simulink model "mA2_vessel"  (R2023a)
settings: Solver=ode4  StartTime=0.0  StopTime=50  FixedStep=0.01  RelTol=1e-3
values from neighbouring files (symbols this model uses):
  B_vessel = 0    [init_mA2_vessel.m]
  d_quay = 0    [init_mA2_vessel.m]
  initial_position = [0,0,0,0,0,0]'    [init_mA2_vessel.m]
  initial_velocity = [0,0,0,0,0,0]'    [init_mA2_vessel.m]
  k_quay = 0    [init_mA2_vessel.m]
  L_vessel = 0    [init_mA2_vessel.m]
  mu_quay = 0    [init_mA2_vessel.m]
  quay_1_depth = 0    [init_mA2_vessel.m]
  quay_1_en = false    [init_mA2_vessel.m]
  quay_1_p0 = [0, 0]'    [init_mA2_vessel.m]
  quay_1_p1 = [0, 0]'    [init_mA2_vessel.m]
  quay_2_depth = 0    [init_mA2_vessel.m]
  quay_2_en = false    [init_mA2_vessel.m]
  quay_2_p0 = [0, 0]'    [init_mA2_vessel.m]
  quay_2_p1 = [0, 0]'    [init_mA2_vessel.m]
  quay_3_depth = 0    [init_mA2_vessel.m]
  quay_3_en = false    [init_mA2_vessel.m]
  quay_3_p0 = [0, 0]'    [init_mA2_vessel.m]
  quay_3_p1 = [0, 0]'    [init_mA2_vessel.m]
  quay_4_depth = 0    [init_mA2_vessel.m]
  quay_4_en = false    [init_mA2_vessel.m]
  quay_4_p0 = [0, 0]'    [init_mA2_vessel.m]
  quay_4_p1 = [0, 0]'    [init_mA2_vessel.m]
libraries: mssSimulink x2
settings Model: Creator=tobiasvt  LastModifiedBy=HalvorPlatou
settings SolverCC: AlgebraicLoopSolver=TrustRegion
settings DebuggingCC: UnconnectedInputMsg=warning  UnconnectedOutputMsg=warning  UnconnectedLineMsg=warning
settings ModelReferenceCC: EnableRefExpFcnMdlSchedulingChecks=on
settings SFSimCC: CustomCodeUndefinedFunction=UseInterfaceOnly
settings RTWCC: Description=FMU based on GRT (Functional Mock-up Unit)  SystemTargetFile=grtfmi.tlc  GenerateMakefile=off  TemplateMakefile=none  RetainRTWFile=on  DLArmComputeVersion=19.05
settings STFCustomTargetCC: ConcurrentExecutionCompliant=off  CombineOutputUpdateFcns=on  CodeInterfacePackaging=Reusable function  GRTInterface=off  GenerateAllocFcn=on  UseToolchainInfoCompliant=off  SystemTargetFile=grtfmi.tlc
settings GRTTargetCC: ParMdlRefBuildCompliant=off  CompOptLevelCompliant=off  ConcurrentExecutionCompliant=off  MatFileLogging=off  CodeInterfacePackaging=Reusable function  CPPClassGenCompliant=off  GenerateAllocFcn=on  UseToolchainInfoCompliant=off

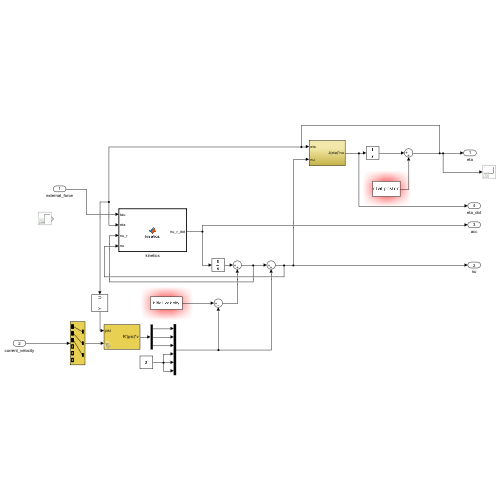
[thumbnail: Simulink's stored preview of the top-level diagram]
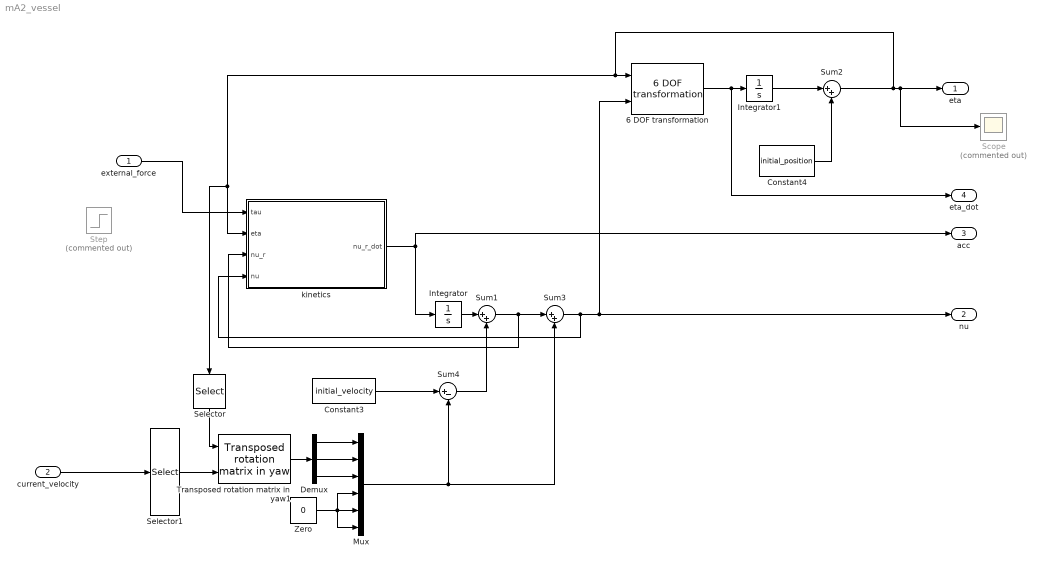
== system mA2_vessel ==
  external_force : Inport  PortDimensions=6
  current_velocity : Inport  Port=2  PortDimensions=6
  6 DOF transformation : mssSimulink/Modelling/Kinematics/6 DOF transformation  SystemSampleTime=-1  VariantActivationTime=update diagram  Latency=0  AutoFrameSizeCalculation=off
  Constant3 : Constant  Value=initial_velocity
  Constant4 : Constant  Value=initial_position
  Demux : Demux  Outputs=3
  Integrator : Integrator
  Integrator1 : Integrator
  Mux : Mux  Inputs=6
  Scope : Scope  Commented=on
  Selector : Selector  InputPortWidth=6  IndexOptions=Index vector (dialog)  Indices=[6]  OutputSizes=1
  Selector1 : Selector  InputPortWidth=6  IndexOptions=Index vector (dialog)  Indices=[1 2 3]  OutputSizes=1
  Step : Step  Commented=on  Before=[0,0,0,0,0,0]  After=[1000,0,0,0,0,0]  SampleTime=0
  Sum1 : Sum  Inputs=|++
  Sum2 : Sum  Inputs=|++
  Sum3 : Sum  Inputs=|++
  Sum4 : Sum  Inputs=|+-
  Transposed rotation matrix in yaw1 : mssSimulink/Modelling/Kinematics/Transposed rotation  matrix in yaw
  Zero : Constant  Value=0  OutDataTypeStr=Inherit: Inherit via back propagation
  kinetics : MATLAB Function  TreatAsAtomicUnit=on
  eta : Outport  VectorParamsAs1DForOutWhenUnconnected=off
  nu : Outport  Port=2  VectorParamsAs1DForOutWhenUnconnected=off
  acc : Outport  Port=3  VectorParamsAs1DForOutWhenUnconnected=off
  eta_dot : Outport  Port=4  VectorParamsAs1DForOutWhenUnconnected=off
  wires:
  Demux/1 -> Mux/1
  Sum1/1 -> kinetics/3(nu_r), Sum3/1
  Demux/3 -> Mux/3
  Selector1/1 -> Transposed rotation matrix in yaw1/2
  Sum2/1 -> 6 DOF transformation/1, Selector/1, kinetics/2(eta), Scope/1, eta/1
  Mux/1 -> Sum4/2, Sum3/2
  Demux/2 -> Mux/2
  kinetics/1(nu_r_dot) -> acc/1, Integrator/1
  Transposed rotation matrix in yaw1/1 -> Demux/1
  Integrator/1 -> Sum1/1
  Zero/1 -> Mux/6, Mux/4, Mux/5
  Constant4/1 -> Sum2/2
  Sum3/1 -> kinetics/4(nu), 6 DOF transformation/2, nu/1
  Selector/1 -> Transposed rotation matrix in yaw1/1
  Integrator1/1 -> Sum2/1
  Constant3/1 -> Sum4/1
  Sum4/1 -> Sum1/2
  6 DOF transformation/1 -> eta_dot/1, Integrator1/1
  current_velocity/1 -> Selector1/1
  external_force/1 -> kinetics/1(tau)

== matlab function mA2_vessel/kinetics ==
  data: tau input; eta input; nu_r_dot output; nu_r input; nu input; mu_quay parameter; d_quay parameter; k_quay parameter; B_vessel parameter; L_vessel parameter; quay_1_en parameter; quay_1_depth parameter; quay_1_p1 parameter; quay_1_p0 parameter; quay_2_en parameter; quay_2_depth parameter; quay_2_p1 parameter; quay_2_p0 parameter; quay_3_en parameter; quay_3_depth parameter; quay_3_p1 parameter; quay_3_p0 parameter; quay_4_en parameter; quay_4_depth parameter; quay_4_p1 parameter; quay_4_p0 parameter
function nu_r_dot  = kinetics(tau, eta, nu_r, nu, mu_quay, d_quay, k_quay, B_vessel, L_vessel, quay_1_en, quay_1_depth, quay_1_p1, quay_1_p0, quay_2_en, quay_2_depth, quay_2_p1, quay_2_p0, quay_3_en, quay_3_depth, quay_3_p1, quay_3_p0, quay_4_en, quay_4_depth, quay_4_p1, quay_4_p0)
% Construct quay parameters
num_quays = sum([quay_1_en, quay_2_en, quay_3_en, quay_4_en]);
s = struct('line', {nan(2, 2)}, 'depth', {nan});
quays = repmat(s,1,num_quays);

i = 1;

if quay_1_en
    quays(i).line = [reshape(quay_1_p0,2,1), reshape(quay_1_p1,2,1)];
    quays(i).depth = quay_1_depth;
    i = i+1;
end
if quay_2_en
    quays(i).line = [reshape(quay_2_p0,2,1), reshape(quay_2_p1,2,1)];
    quays(i).depth = quay_2_depth;
    i = i+1;
end
if quay_3_en
    quays(i).line = [reshape(quay_3_p0,2,1), reshape(quay_3_p1,2,1)];
    quays(i).depth = quay_3_depth;
    i = i+1;
end
if quay_4_en
    quays(i).line = [reshape(quay_4_p0,2,1), reshape(quay_4_p1,2,1)];
    quays(i).depth = quay_4_depth;
    i = i+1;
end

par.mu = mu_quay;
par.k = k_quay;
par.d = d_quay;
par.v_static = 0.1;
par.stiction_damping = true;
par.vessel_polygon = [
    [L_vessel/2, B_vessel/2]
    [L_vessel/2, -B_vessel/2]
    [-L_vessel/2, -B_vessel/2]
    [-L_vessel/2, B_vessel/2]
]';

% Kinetics
u = nu_r(1);
v = nu_r(2);
r = nu_r(6);

%% Horizontal kinetics
%Hydrodynamic coefficients
m_11 = 6.8919e+03;
m_22 = 7.0591e+03;
m_33 = 3.8634e+04;
X_u = -238.5842;
X_auu = -37.1570;
X_uuu = -50.4657;
Y_v = -65.8904;
Y_avv = -300.3485;
Y_vvv = -1.8040;
Y_arv = -4.3745e+03;
Y_r = 232.5028;
Y_avr = 1.4092e+03;
Y_arr = -948.7467;
Y_ur = 223.7115;
N_v = 27.2702;
N_avv = -12.5495;
N_arv = 2.0957e+03;
N_r = -880.0850;
N_arr = -6.6088e+03;
N_avr = -583.9914;
N_uv = -262.3232;
N_ur = 854.4464;

%Mass matrix
M = [m_11 0.0 0.0;
    0.0 m_22 0.0;
    0.0 0.0 m_33];

%Damping matrix
d_11 = -X_u - X_auu*abs(u) - X_uuu*u^2;
d_22 = -Y_v - Y_avv*abs(v) - Y_arv*abs(r) - Y_vvv*v^2;
d_23 = -Y_r - Y_avr*abs(v) - Y_arr*abs(r) - Y_ur*u;
d_32 = -N_v - N_avv*abs(v) - N_arv*abs(r) - N_uv*u;
d_33 = -N_r - N_avr*abs(v) - N_arr*abs(r) - N_ur*u;

D = [d_11, 0, 0;
    0, d_22, d_23;
    0, d_32, d_33];

%Coriolis matrix
c_13 =  -m_22*v;
c_23 =  m_11*u;
c_31 = -c_13;
c_32 = -c_23;

C = [0, 0, c_13;
    0, 0, c_23;
    c_31, c_32, 0];
tau_hor = (-(D + C)*[u,v,r]' + tau([1 2 6]));

tau_quay = quay_tau(eta, nu, [tau_hor(1), tau_hor(2), 0, 0, 0, tau_hor(3)], quays, par);
nu_dot_hor = M\(tau_hor + tau_quay([1,2,6]));

%% Vertical kinetics
%Damping ratios
zeta_heave = 0.1;
zeta_roll = 0.1;
zeta_pitch = 0.1;

Zeta = diag([zeta_heave, zeta_roll, zeta_pitch]);

%Natural periods
T_heave = 1.0;
T_roll = 1.0;
T_pitch = 2.0;
Omega = diag([2*pi/T_heave, 2*pi/T_roll, 2*pi/T_pitch]);

%Inertias (including added mass)
% Calculated assuming moment of inertia is for a uniform rectangle and
% added mass = actual mass -> m_33 = 2*m, m_44 = 2*I_44, m_55 = 2*I_55
m_33 = 9614;
m_44 = 1.8721e+04;
m_55 = 5.6608e+04;
M_vert = diag([m_33, m_44, m_55]);

nu_vert = nu_r([3,4,5]);
eta_vert = eta([3,4,5]);
tau_vert = tau([3,4,5]);

nu_dot_vert = -2*Zeta*Omega*nu_vert - Omega^2*eta_vert + M_vert\tau_vert;


nu_r_dot = [nu_dot_hor(1), nu_dot_hor(2) nu_dot_vert(1) ...
        nu_dot_vert(2), nu_dot_vert(3), nu_dot_hor(3)]';

end
